simulink model "different_inverter_controls_BPS"  (R2024b)
settings: Solver=ode4  StartTime=0.0  StopTime=5  FixedStep=Ts  RelTol=1e-3
InitFcn:
  | %mode_of_operation=1;
  | %BESS_control_mode=1;
  | %Gen_Q_Control =1;
  | 
  | %Exciter_init;
  | 
  | %Exciter_init
  | Xq=0.474;
  | %%====================================================
  | % ST6C Exciter Parameters
  | 
  | KPA=30;
  | KIA=59.91;
  | KFF=1;
  | KM=1;
  | KLR=22.47;
  | KCL=1.04;
  | VAMAX=7.05;
  | VAMIN=-6.11;
  | VRMAX=7.05;
  | VRMIN=-6.11;
  | ILR=5.02;
  | KG=1;
  | TG=0.024;
  | TA=0.01;
  | VBMAX=999;
  | VMMAX=7.05;
  | VMMIN=-6.11;
  | KI=0;
  | Kp=1;
  | Kc=0;
  | Vt0=0;
  | VAAMAX=VAMAX;
  | %%========================================================
  | % UEL2C parameters
  | 
  | TUQ=.005;
  | TUP=0.050;
  | TUV=0.2;
  | TQREF=0;
  | Tadj=0;
  | K1=0;
  | K2=2;
  | VBIAS=1;
  | KFB=0;
  | TUL=0;
  | VUImax=1;
  | VUImin=-1;
  | VUELmax1=1;
  | VUELmax2=1;
  | VUELmin1=-1;
  | VUELmin2=-1;
  | KUF=0;
  | KUL=0.24;
  | KUI=0.001;
  | TU1=0;TU2=0;TU3=0;TU4=0;
  | KFIX=1;
  | VF=0;
  | VFB=0;
  | %%===========================================================
  | ... (+60 lines)
values from neighbouring files (symbols this model uses):
  inv1 = struct    [multiInverterParams.m]
  kp_sync = KQ_p/10    (= 0.04)    [multiInverterParams.m]
  Vdc = 1000    [multiInverterParams.m]
  Vpp = 480    [multiInverterParams.m]
undefined symbols (not defined in the file or in its folder): D1, Delta, DiscIntNeverNeededParam, Ion, Lithium, sigbuilder_block, sps
libraries: slpidlib x34, spsThreePhaseVIMeasurementLib x31, spsThreePhaseSeriesRLCBranchLib x23, spsabctodq0Lib x22, spsPower3phInstantaneousLib x22, spsThreePhaseTransformerTwoWindingsLib x16, spsSeriesRLCBranchLib x16, spsThreePhaseSeriesRLCLoadLib x14, simulink x12, spsPLL3phLib x11, spsGroundLib x9, powerlib_extras x8
(part 9 of 9)

== system different_inverter_controls_BPS/IBR-GFM Power Synchronization/Inverter/Power Controller/P,Q Control /Integrator1 ==
  w : Inport
  Constant1 : Constant  Commented=on  Value=2*pi  SampleTime=Ts
  Constant2 : Constant  Value=2*pi  SampleTime=Ts_Control
  Constant3 : Constant  Commented=on  Value=2*pi  SampleTime=Ts
  Constant4 : Constant  Commented=on  Value=f  SampleTime=Ts_Control
  Constant5 : Constant  Commented=on  Value=0  SampleTime=Ts_Control
  Discrete-Time Integrator : DiscreteIntegrator  Commented=on  IntegratorMethod=Integration: Trapezoidal  SampleTime=Ts  ICPrevOutput=DiscIntNeverNeededParam  ICPrevScaledInput=DiscIntNeverNeededParam
  Discrete-Time Integrator1 : DiscreteIntegrator  ExternalReset=rising  InitialConditionSource=external  SampleTime=Ts_Control  ShowStatePort=on  ICPrevOutput=DiscIntNeverNeededParam  ICPrevScaledInput=DiscIntNeverNeededParam
  Divide : Product  Commented=on  Inputs=*/
  From : From  Commented=on  GotoTag=fsys
  Gain : Gain  Commented=on  Gain=2*pi*f
  Gain1 : Gain  Commented=on  Gain=2*pi*f  SaturateOnIntegerOverflow=on  OutDataTypeStr=Inherit: Same as input  ParamDataTypeStr=Inherit: Same as input
  Gain3 : Gain  Gain=2*pi*f
  Hit Crossing : HitCross  Commented=on  HitCrossingOffset=pi  HitCrossingDirection=falling  ShowOutputPort=off
  Initial : InitialCondition  Value=0
  Initial1 : InitialCondition  Commented=on  Value=0
  Integrator : Integrator  Commented=on  ExternalReset=rising  InitialConditionSource=external  InitialCondition=sps.Phase_Init*pi/180  LimitOutput=on  ShowStatePort=on
  Integrator2 : Integrator  Commented=on  ExternalReset=rising  InitialConditionSource=external  InitialCondition=sps.Phase_Init*pi/180  ShowStatePort=on
  Math Function : Math  Commented=on  Operator=mod  SignedPower=on
  Relational Operator : RelationalOperator  Operator=>  OutDataTypeStr=boolean  InputSameDT=off
  Relational Operator1 : RelationalOperator  Commented=on  Operator=>  OutDataTypeStr=boolean  InputSameDT=off
  Scope : Scope
  Scope1 : Scope  Commented=on
  Scope2 : Scope  Commented=on
  Scope3 : Scope  Commented=on
  Subtract : Sum  Inputs=+-
  Subtract1 : Sum  Commented=on  Inputs=+-
  Sum1 : Sum  Commented=on  Inputs=|++
  Sum2 : Sum  Commented=on  Inputs=|+-
  Theta : Outport
  wires:
  Divide/1 -> Sum1/2
  Constant4/1 -> Divide/2
  From/1 -> Divide/1
  Sum2/1 -> Sum1/1, Scope2/1  "W"
  Constant5/1 -> Sum2/2
  Sum1/1 -> Gain/1  "W"
  Math Function/1 -> Scope1/1
  Constant3/1 -> Math Function/2
  Discrete-Time Integrator/1 -> Math Function/1
  Gain/1 -> Discrete-Time Integrator/1
  Discrete-Time Integrator1/1 -> Theta/1, Scope/1
  Subtract/1 -> Initial/1
  Constant2/1 -> Relational Operator/2, Subtract/2
  Discrete-Time Integrator1/State -> Relational Operator/1, Subtract/1
  Initial/1 -> Discrete-Time Integrator1/3
  Relational Operator/1 -> Discrete-Time Integrator1/2
  Subtract1/1 -> Initial1/1
  Integrator/1 -> Hit Crossing/1, Scope3/1
  Constant1/1 -> Relational Operator1/2, Subtract1/2
  Integrator/State -> Relational Operator1/1, Subtract1/1
  Relational Operator1/1 -> Integrator/2
  Initial1/1 -> Integrator/3
  Gain1/1 -> Integrator/1
  w/1 -> Gain3/1, Sum2/1
  Gain3/1 -> Discrete-Time Integrator1/1

== system different_inverter_controls_BPS/IBR-GFM Power Synchronization/Inverter/Power Controller/P,Q Control /Integrator2 ==
  w : Inport
  Constant1 : Constant  Commented=on  Value=2*pi  SampleTime=Ts
  Constant2 : Constant  Value=2*pi  SampleTime=Ts_Control
  Constant3 : Constant  Commented=on  Value=2*pi  SampleTime=Ts
  Constant4 : Constant  Commented=on  Value=f  SampleTime=Ts_Control
  Constant5 : Constant  Commented=on  Value=0  SampleTime=Ts_Control
  Discrete-Time Integrator : DiscreteIntegrator  Commented=on  IntegratorMethod=Integration: Trapezoidal  SampleTime=Ts  ICPrevOutput=DiscIntNeverNeededParam  ICPrevScaledInput=DiscIntNeverNeededParam
  Discrete-Time Integrator1 : DiscreteIntegrator  ExternalReset=rising  InitialConditionSource=external  SampleTime=Ts_Control  ShowStatePort=on  ICPrevOutput=DiscIntNeverNeededParam  ICPrevScaledInput=DiscIntNeverNeededParam
  Divide : Product  Commented=on  Inputs=*/
  From : From  Commented=on  GotoTag=fsys
  Gain : Gain  Commented=on  Gain=2*pi*f
  Gain1 : Gain  Commented=on  Gain=2*pi*f  SaturateOnIntegerOverflow=on  OutDataTypeStr=Inherit: Same as input  ParamDataTypeStr=Inherit: Same as input
  Gain3 : Gain  Gain=2*pi*f
  Hit Crossing : HitCross  Commented=on  HitCrossingOffset=pi  HitCrossingDirection=falling  ShowOutputPort=off
  Initial : InitialCondition  Value=0
  Initial1 : InitialCondition  Commented=on  Value=0
  Integrator : Integrator  Commented=on  ExternalReset=rising  InitialConditionSource=external  InitialCondition=sps.Phase_Init*pi/180  LimitOutput=on  ShowStatePort=on
  Integrator2 : Integrator  Commented=on  ExternalReset=rising  InitialConditionSource=external  InitialCondition=sps.Phase_Init*pi/180  ShowStatePort=on
  Math Function : Math  Commented=on  Operator=mod  SignedPower=on
  Relational Operator : RelationalOperator  Operator=>  OutDataTypeStr=boolean  InputSameDT=off
  Relational Operator1 : RelationalOperator  Commented=on  Operator=>  OutDataTypeStr=boolean  InputSameDT=off
  Scope : Scope
  Scope1 : Scope  Commented=on
  Scope2 : Scope  Commented=on
  Scope3 : Scope  Commented=on
  Subtract : Sum  Inputs=+-
  Subtract1 : Sum  Commented=on  Inputs=+-
  Sum1 : Sum  Commented=on  Inputs=|++
  Sum2 : Sum  Commented=on  Inputs=|+-
  Theta : Outport
  wires:
  Gain3/1 -> Discrete-Time Integrator1/1
  w/1 -> Sum2/1, Gain3/1
  Gain1/1 -> Integrator/1
  Initial1/1 -> Integrator/3
  Relational Operator1/1 -> Integrator/2
  Integrator/State -> Subtract1/1, Relational Operator1/1
  Constant1/1 -> Subtract1/2, Relational Operator1/2
  Integrator/1 -> Scope3/1, Hit Crossing/1
  Subtract1/1 -> Initial1/1
  Relational Operator/1 -> Discrete-Time Integrator1/2
  Initial/1 -> Discrete-Time Integrator1/3
  Discrete-Time Integrator1/State -> Subtract/1, Relational Operator/1
  Constant2/1 -> Subtract/2, Relational Operator/2
  Subtract/1 -> Initial/1
  Discrete-Time Integrator1/1 -> Scope/1, Theta/1
  Gain/1 -> Discrete-Time Integrator/1
  Discrete-Time Integrator/1 -> Math Function/1
  Constant3/1 -> Math Function/2
  Math Function/1 -> Scope1/1
  Sum1/1 -> Gain/1  "W"
  Constant5/1 -> Sum2/2
  Sum2/1 -> Scope2/1, Sum1/1  "W"
  From/1 -> Divide/1
  Constant4/1 -> Divide/2
  Divide/1 -> Sum1/2

== system different_inverter_controls_BPS/GFM-VSG-100MW/IBR-GFM VSG/Inverter/Inverter Control/Current Control/Current Regulator ==
  note: Current Regulator
      | ================
  note: Sign Convention: Current going out of the converter = positive current
  note: Iq positive --> The converter absorbs reactive power ("Inductive mode") = Reactive Power Q negative
  note: Id positive --> The converter generates active power ("Inverter mode") = Active Power P positive
  VdVq_meas : Inport  PortDimensions=2
  IdIq_meas : Inport  Port=2  PortDimensions=2
  IdIq_ref : Inport  Port=3  PortDimensions=2
  Add1 : Sum  Inputs=++-
  Add2 : Sum
  Add3 : Sum  Inputs=+++
  Demux : Demux  Outputs=2
  Demux1 : Demux  Outputs=2
  Lff : Gain  Gain=inv1.Lpu  SaturateOnIntegerOverflow=on  OutDataTypeStr=Inherit: Same as input  ParamDataTypeStr=Inherit: Same as input
  "Lff  " : Gain  Gain=inv1.Lpu  SaturateOnIntegerOverflow=on  OutDataTypeStr=Inherit: Same as input  ParamDataTypeStr=Inherit: Same as input
  Lff  1 : Gain  Commented=on  Gain=Ltot_pu  SaturateOnIntegerOverflow=on  OutDataTypeStr=Inherit: Same as input  ParamDataTypeStr=Inherit: Same as input
  Mux : Mux  Inputs=2
  PI : slpidlib/PID Controller  Controller=PI  Form=Parallel  TimeDomain=Discrete-time  UseExternalTs=off  SampleTime=Ts_Control  IntegratorMethod=Forward Euler  FilterMethod=Forward Euler  ControllerParametersSource=internal  P=Kp_Ireg/10  I=Ki_Ireg  UseKiTs=off  D=0  UseExternalDerivativeSource=off  N=100  UseFilter=on  TunerSelectOption=Transfer Function Based (PID Tuner App)  InitialConditionSource=internal  InitialConditionForIntegrator=0  InitialConditionForFilter=0  DifferentiatorICPrevScaledInput=0  ExternalReset=none  TrackingMode=off  Kt=1  LimitOutput=on  SatLimitsSource=internal  UpperSaturationLimit=1.5  LowerSaturationLimit=-1.5  LinearizeAsGain=off  AntiWindupMode=back-calculation  Kb=1  LimitIntegrator=off  UpperIntegratorSaturationLimit=inf  LowerIntegratorSaturationLimit=-inf  POutMin=[]  POutMax=[]  IOutMin=[]  IOutMax=[]  DOutMin=[]  DOutMax=[]  NOutMin=[]  NOutMax=[]  SumOutMin=[]  SumOutMax=[]  SaturationOutMin=[]  SaturationOutMax=[]  PParamMin=[]  PParamMax=[]  IParamMin=[]  IParamMax=[]  DParamMin=[]  DParamMax=[]  NParamMin=[]  NParamMax=[]  KbParamMin=[]  KbParamMax=[]  KtParamMin=[]  KtParamMax=[]  KbOutMin=[]  KbOutMax=[]  KtOutMin=[]  KtOutMax=[]  IntegratorOutMin=[]  IntegratorOutMax=[]  FilterOutMin=[]  FilterOutMax=[]  SumI1OutMin=[]  SumI1OutMax=[]  SumI2OutMin=[]  SumI2OutMax=[]  SumI3OutMin=[]  SumI3OutMax=[]  SumI4OutMin=[]  SumI4OutMax=[]  SumDOutMin=[]  SumDOutMax=[]  DifferentiatorOutMin=[]  DifferentiatorOutMax=[]  FilterDiffOutCoefMin=[]  FilterDiffOutCoefMax=[]  ReciprocalOutMin=[]  ReciprocalOutMax=[]  SumDenOutMin=[]  SumDenOutMax=[]  SumNumOutMin=[]  SumNumOutMax=[]  DivideOutMin=[]  DivideOutMax=[]  UdiffTsProdOutMin=[]  UdiffTsProdOutMax=[]  NTsProdOutMin=[]  NTsProdOutMax=[]  UintegralTsProdOutMin=[]  UintegralTsProdOutMax=[]  UngainTsProdOutMin=[]  UngainTsProdOutMax=[]  ClampingZeroOutDataTypeStr=Inherit: Inherit via back propagation  ClampingZeroOutMin=[]  ClampingZeroOutMax=[]  FilterDenConstantOutDataTypeStr=Inherit: Inherit via back propagation  FilterDenConstantOutMin=[]  FilterDenConstantOutMax=[]  PCopyOutDataTypeStr=Inherit: Inherit via back propagation  PCopyOutMin=[]  PCopyOutMax=[]  NCopyOutDataTypeStr=Inherit: Inherit via back propagation  NCopyOutMin=[]  NCopyOutMax=[]  IntegratorContinuousStateAttributes=''  IntegratorStateMustResolveToSignalObject=off  IntegratorRTWStateStorageClass=Auto  FilterContinuousStateAttributes=''  FilterStateMustResolveToSignalObject=off  FilterRTWStateStorageClass=Auto  ParallelPVariant=InternalParameters  IdealPVariant=Disabled  IVariant=InternalParameters  DVariant=Disabled  IntegratorVariant=Discrete  SatVariant=Enabled  AWVariant=BackCalculation  PCopyVariant=Disabled  TRVariant=Disabled  FdbkBlocksVariant=Forward  IdealPFdbkVariant=Disabled  SatFdbkVariant=Disabled  DerivativeFilterVariant=Disabled  NVariant=Disabled  NCopyVariant=Disabled_SignalSpec  FilterICVariant=Disabled  IntegratorICVariant=InternalICs  ExternalResetVariant=Disabled  TRSumVariant=Passthrough  SumFdbkVariant=Disabled  SumVariant=Sum_PI  TsampFilterVariant=InternalTs  TsampNgainVariant=Passthrough  TsampIntegralVariant=Disabled_SignalSpec  ExternalSaturationOutDataTypeStr=Inherit: Same as second input  DerivativeSourceVariant=Disabled  PreIntVariant=InternalPreInt
  PI1 : slpidlib/PID Controller  Commented=on  Controller=PI  Form=Parallel  TimeDomain=Discrete-time  UseExternalTs=off  SampleTime=Ts_Control  IntegratorMethod=Forward Euler  FilterMethod=Forward Euler  ControllerParametersSource=internal  P=Kp_Ireg  I=Ki_Ireg  UseKiTs=off  D=0  UseExternalDerivativeSource=off  N=100  UseFilter=on  TunerSelectOption=Transfer Function Based (PID Tuner App)  InitialConditionSource=internal  InitialConditionForIntegrator=0  InitialConditionForFilter=0  DifferentiatorICPrevScaledInput=0  ExternalReset=none  TrackingMode=off  Kt=1  LimitOutput=on  SatLimitsSource=internal  UpperSaturationLimit=1.5  LowerSaturationLimit=-1.5  LinearizeAsGain=off  AntiWindupMode=clamping  Kb=1  LimitIntegrator=off  UpperIntegratorSaturationLimit=inf  LowerIntegratorSaturationLimit=-inf  POutMin=[]  POutMax=[]  IOutMin=[]  IOutMax=[]  DOutMin=[]  DOutMax=[]  NOutMin=[]  NOutMax=[]  SumOutMin=[]  SumOutMax=[]  SaturationOutMin=[]  SaturationOutMax=[]  PParamMin=[]  PParamMax=[]  IParamMin=[]  IParamMax=[]  DParamMin=[]  DParamMax=[]  NParamMin=[]  NParamMax=[]  KbParamMin=[]  KbParamMax=[]  KtParamMin=[]  KtParamMax=[]  KbOutMin=[]  KbOutMax=[]  KtOutMin=[]  KtOutMax=[]  IntegratorOutMin=[]  IntegratorOutMax=[]  FilterOutMin=[]  FilterOutMax=[]  SumI1OutMin=[]  SumI1OutMax=[]  SumI2OutMin=[]  SumI2OutMax=[]  SumI3OutMin=[]  SumI3OutMax=[]  SumI4OutMin=[]  SumI4OutMax=[]  SumDOutMin=[]  SumDOutMax=[]  DifferentiatorOutMin=[]  DifferentiatorOutMax=[]  FilterDiffOutCoefMin=[]  FilterDiffOutCoefMax=[]  ReciprocalOutMin=[]  ReciprocalOutMax=[]  SumDenOutMin=[]  SumDenOutMax=[]  SumNumOutMin=[]  SumNumOutMax=[]  DivideOutMin=[]  DivideOutMax=[]  UdiffTsProdOutMin=[]  UdiffTsProdOutMax=[]  NTsProdOutMin=[]  NTsProdOutMax=[]  UintegralTsProdOutMin=[]  UintegralTsProdOutMax=[]  UngainTsProdOutMin=[]  UngainTsProdOutMax=[]  ClampingZeroOutDataTypeStr=Inherit: Inherit via back propagation  ClampingZeroOutMin=[]  ClampingZeroOutMax=[]  FilterDenConstantOutDataTypeStr=Inherit: Inherit via back propagation  FilterDenConstantOutMin=[]  FilterDenConstantOutMax=[]  PCopyOutDataTypeStr=Inherit: Inherit via back propagation  PCopyOutMin=[]  PCopyOutMax=[]  NCopyOutDataTypeStr=Inherit: Inherit via back propagation  NCopyOutMin=[]  NCopyOutMax=[]  IntegratorContinuousStateAttributes=''  IntegratorStateMustResolveToSignalObject=off  IntegratorRTWStateStorageClass=Auto  FilterContinuousStateAttributes=''  FilterStateMustResolveToSignalObject=off  FilterRTWStateStorageClass=Auto  ParallelPVariant=InternalParameters  IdealPVariant=Disabled  IVariant=InternalParameters  DVariant=Disabled  IntegratorVariant=Discrete  SatVariant=Enabled  AWVariant=DiscClampingParallel  PCopyVariant=Disabled  TRVariant=Disabled  FdbkBlocksVariant=Forward  IdealPFdbkVariant=Disabled  SatFdbkVariant=Disabled  DerivativeFilterVariant=Disabled  NVariant=Disabled  NCopyVariant=Disabled_SignalSpec  FilterICVariant=Disabled  IntegratorICVariant=InternalICs  ExternalResetVariant=Disabled  TRSumVariant=Passthrough  SumFdbkVariant=Disabled  SumVariant=Sum_PI  TsampFilterVariant=InternalTs  TsampNgainVariant=Passthrough  TsampIntegralVariant=Disabled_SignalSpec  ExternalSaturationOutDataTypeStr=Inherit: Same as second input  DerivativeSourceVariant=Disabled  PreIntVariant=InternalPreInt
  PI2 : slpidlib/PID Controller  Commented=on  Controller=PI  Form=Parallel  TimeDomain=Discrete-time  UseExternalTs=off  SampleTime=Ts_Control  IntegratorMethod=Forward Euler  FilterMethod=Forward Euler  ControllerParametersSource=internal  P=Kp_Ireg  I=Ki_Ireg  UseKiTs=off  D=0  UseExternalDerivativeSource=off  N=100  UseFilter=on  TunerSelectOption=Transfer Function Based (PID Tuner App)  InitialConditionSource=internal  InitialConditionForIntegrator=0  InitialConditionForFilter=0  DifferentiatorICPrevScaledInput=0  ExternalReset=none  TrackingMode=off  Kt=1  LimitOutput=on  SatLimitsSource=internal  UpperSaturationLimit=1.5  LowerSaturationLimit=-1.5  LinearizeAsGain=off  AntiWindupMode=back-calculation  Kb=1  LimitIntegrator=off  UpperIntegratorSaturationLimit=inf  LowerIntegratorSaturationLimit=-inf  POutMin=[]  POutMax=[]  IOutMin=[]  IOutMax=[]  DOutMin=[]  DOutMax=[]  NOutMin=[]  NOutMax=[]  SumOutMin=[]  SumOutMax=[]  SaturationOutMin=[]  SaturationOutMax=[]  PParamMin=[]  PParamMax=[]  IParamMin=[]  IParamMax=[]  DParamMin=[]  DParamMax=[]  NParamMin=[]  NParamMax=[]  KbParamMin=[]  KbParamMax=[]  KtParamMin=[]  KtParamMax=[]  KbOutMin=[]  KbOutMax=[]  KtOutMin=[]  KtOutMax=[]  IntegratorOutMin=[]  IntegratorOutMax=[]  FilterOutMin=[]  FilterOutMax=[]  SumI1OutMin=[]  SumI1OutMax=[]  SumI2OutMin=[]  SumI2OutMax=[]  SumI3OutMin=[]  SumI3OutMax=[]  SumI4OutMin=[]  SumI4OutMax=[]  SumDOutMin=[]  SumDOutMax=[]  DifferentiatorOutMin=[]  DifferentiatorOutMax=[]  FilterDiffOutCoefMin=[]  FilterDiffOutCoefMax=[]  ReciprocalOutMin=[]  ReciprocalOutMax=[]  SumDenOutMin=[]  SumDenOutMax=[]  SumNumOutMin=[]  SumNumOutMax=[]  DivideOutMin=[]  DivideOutMax=[]  UdiffTsProdOutMin=[]  UdiffTsProdOutMax=[]  NTsProdOutMin=[]  NTsProdOutMax=[]  UintegralTsProdOutMin=[]  UintegralTsProdOutMax=[]  UngainTsProdOutMin=[]  UngainTsProdOutMax=[]  ClampingZeroOutDataTypeStr=Inherit: Inherit via back propagation  ClampingZeroOutMin=[]  ClampingZeroOutMax=[]  FilterDenConstantOutDataTypeStr=Inherit: Inherit via back propagation  FilterDenConstantOutMin=[]  FilterDenConstantOutMax=[]  PCopyOutDataTypeStr=Inherit: Inherit via back propagation  PCopyOutMin=[]  PCopyOutMax=[]  NCopyOutDataTypeStr=Inherit: Inherit via back propagation  NCopyOutMin=[]  NCopyOutMax=[]  IntegratorContinuousStateAttributes=''  IntegratorStateMustResolveToSignalObject=off  IntegratorRTWStateStorageClass=Auto  FilterContinuousStateAttributes=''  FilterStateMustResolveToSignalObject=off  FilterRTWStateStorageClass=Auto  ParallelPVariant=InternalParameters  IdealPVariant=Disabled  IVariant=InternalParameters  DVariant=Disabled  IntegratorVariant=Discrete  SatVariant=Enabled  AWVariant=BackCalculation  PCopyVariant=Disabled  TRVariant=Disabled  FdbkBlocksVariant=Forward  IdealPFdbkVariant=Disabled  SatFdbkVariant=Disabled  DerivativeFilterVariant=Disabled  NVariant=Disabled  NCopyVariant=Disabled_SignalSpec  FilterICVariant=Disabled  IntegratorICVariant=InternalICs  ExternalResetVariant=Disabled  TRSumVariant=Passthrough  SumFdbkVariant=Disabled  SumVariant=Sum_PI  TsampFilterVariant=InternalTs  TsampNgainVariant=Passthrough  TsampIntegralVariant=Disabled_SignalSpec  ExternalSaturationOutDataTypeStr=Inherit: Same as second input  DerivativeSourceVariant=Disabled  PreIntVariant=InternalPreInt
  Rff : Gain  Commented=on  Gain=inv1.R/inv1.Zb  SaturateOnIntegerOverflow=on  OutDataTypeStr=Inherit: Same as input  ParamDataTypeStr=Inherit: Same as input
  "Rff " : Gain  Commented=on  Gain=inv1.R/inv1.Zb  SaturateOnIntegerOverflow=on  OutDataTypeStr=Inherit: Same as input  ParamDataTypeStr=Inherit: Same as input
  Rff 1 : Gain  Commented=on  Gain=Rtot_pu  SaturateOnIntegerOverflow=on  OutDataTypeStr=Inherit: Same as input  ParamDataTypeStr=Inherit: Same as input
  Saturation : Saturate  UpperLimit=1.5  LowerLimit=-1.5
  Scope : Scope  NumInputPorts=2
  Scope1 : Scope
  Sum : Sum  Inputs=|-+
  VdVq_conv : Outport  VectorParamsAs1DForOutWhenUnconnected=off
  wires:
  Mux/1 -> Add2/2
  PI/1 -> Scope/2, Add2/1  "PI"
  Sum/1 -> Scope/1, PI/1
  IdIq_ref/1 -> Sum/2
  IdIq_meas/1 -> Demux1/1, Sum/1
  Add2/1 -> Saturation/1
  Saturation/1 -> Scope1/1, VdVq_conv/1
  VdVq_meas/1 -> Demux/1
  Demux/1 -> Add1/1
  "Rff "/1 -> Add1/2
  Demux1/1 -> "Rff "/1, Lff/1
  "Lff  "/1 -> Add1/3
  Demux1/2 -> "Lff  "/1, Rff/1
  Rff/1 -> Add3/2
  Lff/1 -> Add3/3
  Add1/1 -> Mux/1  "Feedforward"
  Demux/2 -> Add3/1
  Add3/1 -> Mux/2

== system different_inverter_controls_BPS/GFM-VSG-100MW/IBR-GFM VSG/Inverter/Inverter Control/Current Control/Uabc_ref Generation max (m) = 1 ==
  note: (Correction for transformer
      |  D1 connection)
  note: (Correction for delay of Ts_Control)
  note: Uref Generation
      | ==============
  wt : Inport
  VdVq_conv : Inport  Port=2
  Add1 : Sum  Inputs=++++
  Add2 : Sum
  Complex to Magnitude-Angle : ComplexToMagnitudeAngle
  Constant : Constant  Commented=on  Value=-pi/6
  Constant1 : Constant  Commented=on  Value=Vnom_dc
  Constant2 : Constant  Value="[ 0  -2*pi/3  2*pi/3  ]"
  Constant3 : Constant  Commented=on  Value=Vnom_sec*sqrt(2)/sqrt(3)
  Constant4 : Constant  Value=Ts_Control*Fnom*(2*pi)
  Constant5 : Constant  Value=Vdc
  Constant6 : Constant  Value=Vpp*sqrt(2)/sqrt(3)
  Demux1 : Demux  Outputs=2
  Gain1 : Gain  Gain=1/2
  Product : Product  Inputs=*/  RndMeth=Zero
  Product1 : Product  Inputs=*/  RndMeth=Zero
  Product2 : Product  Inputs=**  RndMeth=Zero
  Real-Imag to Complex : RealImagToComplex
  Trigonometric Function : Trigonometry
  Uabc_ref : Outport  VectorParamsAs1DForOutWhenUnconnected=off
  wires:
  Constant5/1 -> Gain1/1
  VdVq_conv/1 -> Product1/1
  Product1/1 -> Demux1/1
  Gain1/1 -> Product/1
  Real-Imag to Complex/1 -> Complex to Magnitude-Angle/1
  Demux1/1 -> Real-Imag to Complex/1
  Demux1/2 -> Real-Imag to Complex/2
  Constant2/1 -> Add1/2
  Constant/1 -> Add1/3
  Constant6/1 -> Product/2
  Complex to Magnitude-Angle/2 -> Add2/1
  Add1/1 -> Add2/2
  Add2/1 -> Trigonometric Function/1
  Complex to Magnitude-Angle/1 -> Product2/1
  Trigonometric Function/1 -> Product2/2
  Product2/1 -> Uabc_ref/1
  wt/1 -> Add1/1
  Constant4/1 -> Add1/4
  Product/1 -> Product1/2

== system different_inverter_controls_BPS/GFM-VSG-100MW/IBR-GFM VSG/Inverter/Inverter Control/current limiter/P priority limit ==
  idiqP : Inport
  Demux4 : Demux  Outputs=2
  IqLimit : Subsystem
  Mux4 : Mux  Inputs=2
  Rtot_pu1 : Gain  Gain=-1  SaturateOnIntegerOverflow=on  OutDataTypeStr=Inherit: Same as input  ParamDataTypeStr=Inherit: Same as input
  Saturation : Saturate  UpperLimit=limMax  LowerLimit=0
  Saturation Dynamic : simulink/Discontinuities/Saturation Dynamic  OutMin=[]  OutMax=[limMax]  OutDataTypeStr=Inherit: Same as second input  OutDataType=fixdt(1, 16)  OutScaling=2^-10  DoSatur=off
  idiqPRefL : Outport
  wires:
  IqLimit/1(Out2) -> Saturation Dynamic/1, Rtot_pu1/1
  Rtot_pu1/1 -> Saturation Dynamic/3
  Saturation/1 -> Mux4/1, IqLimit/1(In1)
  Demux4/1 -> Saturation/1
  Mux4/1 -> idiqPRefL/1
  Demux4/2 -> Saturation Dynamic/2
  idiqP/1 -> Demux4/1
  Saturation Dynamic/1 -> Mux4/2

== system different_inverter_controls_BPS/GFM-VSG-100MW/IBR-GFM VSG/Inverter/Inverter Control/current limiter/Q priority limit ==
  idiqP : Inport
  V_inv_mag : Inport  Port=2
  Demux4 : Demux  Outputs=2
  Iq condition : Switch  Threshold=0.9  SaturateOnIntegerOverflow=off  InputSameDT=off
  IqLimit : Subsystem
  Mux4 : Mux  Inputs=2
  Rtot_pu1 : Gain  Gain=-1  SaturateOnIntegerOverflow=on  OutDataTypeStr=Inherit: Same as input  ParamDataTypeStr=Inherit: Same as input
  Saturation : Saturate  UpperLimit=limMax  LowerLimit=limMin
  Saturation Dynamic : simulink/Discontinuities/Saturation Dynamic  OutMin=[]  OutMax=[]  OutDataTypeStr=Inherit: Same as second input  OutDataType=fixdt(1, 16)  OutScaling=2^-10  DoSatur=off
  Saturation1 : Saturate  UpperLimit=0  LowerLimit=limMin
  Scope : Scope
  idiqPRefL : Outport
  wires:
  Demux4/2 -> Saturation1/1, Saturation/1
  Saturation1/1 -> Iq condition/3
  IqLimit/1(Out2) -> Saturation Dynamic/1, Rtot_pu1/1
  Demux4/1 -> Saturation Dynamic/2
  Saturation Dynamic/1 -> Mux4/1
  Rtot_pu1/1 -> Saturation Dynamic/3
  Mux4/1 -> idiqPRefL/1
  idiqP/1 -> Demux4/1
  Saturation/1 -> Iq condition/1
  V_inv_mag/1 -> Iq condition/2
  Iq condition/1 -> IqLimit/1(In1), Mux4/2

== system different_inverter_controls_BPS/GFM-VSG-100MW/IBR-GFM VSG/Inverter/Inverter Control/current limiter/Subsystem3 ==
  In1 : Inport
  Demux2 : Demux  Outputs=2
  Math Function : Math  Operator=square  SignedPower=on
  Saturation : Saturate  UpperLimit=limMax  LowerLimit=limMin
  Scope : Scope  NumInputPorts=2
  Sqrt1 : Sqrt
  Subtract : Sum
  Out1 : Outport
  Out2 : Outport  Port=2
  wires:
  Saturation/1 -> Out1/1
  Sqrt1/1 -> Out2/1, Scope/1, Saturation/1
  Subtract/1 -> Sqrt1/1  "Ipos2"
  In1/1 -> Math Function/1, Scope/2
  Math Function/1 -> Demux2/1
  Demux2/1 -> Subtract/1
  Demux2/2 -> Subtract/2

== system different_inverter_controls_BPS/GFM-VSG-100MW/IBR-GFM VSG/Inverter/Inverter Control/current limiter/Subsystem4 ==
  In1 : Inport
  In2 : Inport  Port=2
  Demux4 : Demux  Outputs=2
  Mux4 : Mux  Inputs=2
  Switch1 : Switch  Threshold=limMax  SaturateOnIntegerOverflow=off  InputSameDT=off
  Unit Delay2 : UnitDelay  InitialCondition=1  SampleTime=Ts_Control  HasFrameUpgradeWarning=on
  dummy limit : Saturate  UpperLimit=limMax  LowerLimit=limMin
  Out1 : Outport
  wires:
  dummy limit/1 -> Mux4/2
  Demux4/2 -> dummy limit/1
  In2/1 -> Demux4/1, Switch1/3
  In1/1 -> Switch1/2
  Unit Delay2/1 -> Switch1/1
  Switch1/1 -> Unit Delay2/1, Mux4/1, Out1/1

== system different_inverter_controls_BPS/GFM-VSG-100MW/IBR-GFM VSG/Inverter/Inverter Control/current limiter/Subsystem9 ==
  In1 : Inport
  In2 : Inport  Port=2
  Divide : Product  Inputs=*/
  Gain1 : Gain  Gain=limMax
  Saturation : Saturate  UpperLimit=limMax  LowerLimit=limMin
  Switch1 : Switch  Threshold=limMax  SaturateOnIntegerOverflow=off  InputSameDT=off
  idiqPRefL : Outport
  wires:
  Saturation/1 -> idiqPRefL/1
  Switch1/1 -> Saturation/1
  Gain1/1 -> Switch1/1
  Divide/1 -> Gain1/1
  In2/1 -> Switch1/3, Divide/1
  In1/1 -> Switch1/2, Divide/2

== system different_inverter_controls_BPS/GFM-VSG-100MW/IBR-GFM VSG/Inverter/Power Controller/P,Q Control /Integrator ==
  w : Inport
  Constant2 : Constant  Value=2*pi  SampleTime=Ts_Control
  Discrete-Time Integrator1 : DiscreteIntegrator  ExternalReset=rising  InitialConditionSource=external  SampleTime=Ts_Control  ShowStatePort=on  ICPrevOutput=DiscIntNeverNeededParam  ICPrevScaledInput=DiscIntNeverNeededParam
  Gain3 : Gain  Gain=2*pi*f
  Initial : InitialCondition  Value=0
  Relational Operator : RelationalOperator  Operator=>  OutDataTypeStr=boolean  InputSameDT=off
  Scope : Scope
  Subtract : Sum  Inputs=+-
  Theta : Outport
  wires:
  Discrete-Time Integrator1/1 -> Theta/1, Scope/1
  Subtract/1 -> Initial/1
  Constant2/1 -> Relational Operator/2, Subtract/2
  Discrete-Time Integrator1/State -> Relational Operator/1, Subtract/1
  Initial/1 -> Discrete-Time Integrator1/3
  Relational Operator/1 -> Discrete-Time Integrator1/2
  w/1 -> Gain3/1
  Gain3/1 -> Discrete-Time Integrator1/1

== system different_inverter_controls_BPS/IBR GFL-SH/BESS/Inverter Control/current limiter/P priority limit/IqLimit ==
  In1 : Inport
  Math Function : Math  Operator=square  SignedPower=on
  Math Function1 : Math  Operator=square  SignedPower=on
  Sqrt : Sqrt
  Subtract : Sum  Inputs=+-
  Vdc_ref1 : Constant  Value=limMax  SampleTime=Ts_Control
  Out2 : Outport
  wires:
  Math Function1/1 -> Subtract/2
  In1/1 -> Math Function1/1
  Vdc_ref1/1 -> Math Function/1
  Subtract/1 -> Sqrt/1
  Sqrt/1 -> Out2/1
  Math Function/1 -> Subtract/1

== system different_inverter_controls_BPS/IBR GFL-SH/BESS/Inverter Control/current limiter/Q priority limit/IqLimit ==
  In1 : Inport
  Math Function : Math  Operator=square  SignedPower=on
  Math Function1 : Math  Operator=square  SignedPower=on
  Sqrt : Sqrt
  Subtract : Sum  Inputs=+-
  Vdc_ref1 : Constant  Value=limMax  SampleTime=Ts_Control
  Out2 : Outport
  wires:
  Math Function1/1 -> Subtract/2
  In1/1 -> Math Function1/1
  Vdc_ref1/1 -> Math Function/1
  Subtract/1 -> Sqrt/1
  Sqrt/1 -> Out2/1
  Math Function/1 -> Subtract/1

== system different_inverter_controls_BPS/IBR GFL-SH/IBR/Inverter Control/current limiter/P priority limit/IqLimit ==
  In1 : Inport
  Math Function : Math  Operator=square  SignedPower=on
  Math Function1 : Math  Operator=square  SignedPower=on
  Sqrt : Sqrt
  Subtract : Sum  Inputs=+-
  Vdc_ref1 : Constant  Value=limMax  SampleTime=Ts_Control
  Out2 : Outport
  wires:
  Math Function1/1 -> Subtract/2
  In1/1 -> Math Function1/1
  Vdc_ref1/1 -> Math Function/1
  Subtract/1 -> Sqrt/1
  Sqrt/1 -> Out2/1
  Math Function/1 -> Subtract/1

== system different_inverter_controls_BPS/IBR GFL-SH/IBR/Inverter Control/current limiter/Q priority limit/IqLimit ==
  In1 : Inport
  Math Function : Math  Operator=square  SignedPower=on
  Math Function1 : Math  Operator=square  SignedPower=on
  Sqrt : Sqrt
  Subtract : Sum  Inputs=+-
  Vdc_ref1 : Constant  Value=limMax  SampleTime=Ts_Control
  Out2 : Outport
  wires:
  Math Function1/1 -> Subtract/2
  In1/1 -> Math Function1/1
  Vdc_ref1/1 -> Math Function/1
  Subtract/1 -> Sqrt/1
  Sqrt/1 -> Out2/1
  Math Function/1 -> Subtract/1

== system different_inverter_controls_BPS/IBR-GFM PV Droop/IBR/Inverter Control/current limiter/P priority limit/IqLimit ==
  In1 : Inport
  Math Function : Math  Operator=square  SignedPower=on
  Math Function1 : Math  Operator=square  SignedPower=on
  Sqrt : Sqrt
  Subtract : Sum  Inputs=+-
  Vdc_ref1 : Constant  Value=limMax  SampleTime=Ts_Control
  Out2 : Outport
  wires:
  Math Function1/1 -> Subtract/2
  In1/1 -> Math Function1/1
  Vdc_ref1/1 -> Math Function/1
  Subtract/1 -> Sqrt/1
  Sqrt/1 -> Out2/1
  Math Function/1 -> Subtract/1

== system different_inverter_controls_BPS/IBR-GFM PV Droop/IBR/Inverter Control/current limiter/Q priority limit/IqLimit ==
  In1 : Inport
  Math Function : Math  Operator=square  SignedPower=on
  Math Function1 : Math  Operator=square  SignedPower=on
  Sqrt : Sqrt
  Subtract : Sum  Inputs=+-
  Vdc_ref1 : Constant  Value=limMax  SampleTime=Ts_Control
  Out2 : Outport
  wires:
  Math Function1/1 -> Subtract/2
  In1/1 -> Math Function1/1
  Vdc_ref1/1 -> Math Function/1
  Subtract/1 -> Sqrt/1
  Sqrt/1 -> Out2/1
  Math Function/1 -> Subtract/1

== system different_inverter_controls_BPS/IBR-GFM Synchro-inverter/Inverter/Inverter Control/current limiter/P priority limit/IqLimit ==
  In1 : Inport
  Math Function : Math  Operator=square  SignedPower=on
  Math Function1 : Math  Operator=square  SignedPower=on
  Sqrt : Sqrt
  Subtract : Sum  Inputs=+-
  Vdc_ref1 : Constant  Value=limMax  SampleTime=Ts_Control
  Out2 : Outport
  wires:
  Math Function/1 -> Subtract/1
  Sqrt/1 -> Out2/1
  Subtract/1 -> Sqrt/1
  Vdc_ref1/1 -> Math Function/1
  In1/1 -> Math Function1/1
  Math Function1/1 -> Subtract/2

== system different_inverter_controls_BPS/IBR-GFM Synchro-inverter/Inverter/Inverter Control/current limiter/Q priority limit/IqLimit ==
  In1 : Inport
  Math Function : Math  Operator=square  SignedPower=on
  Math Function1 : Math  Operator=square  SignedPower=on
  Sqrt : Sqrt
  Subtract : Sum  Inputs=+-
  Vdc_ref1 : Constant  Value=limMax  SampleTime=Ts_Control
  Out2 : Outport
  wires:
  Math Function/1 -> Subtract/1
  Sqrt/1 -> Out2/1
  Subtract/1 -> Sqrt/1
  Vdc_ref1/1 -> Math Function/1
  In1/1 -> Math Function1/1
  Math Function1/1 -> Subtract/2

== system different_inverter_controls_BPS/IBR-GFM Power Synchronization/Inverter/Inverter Control/current limiter/P priority limit/IqLimit ==
  In1 : Inport
  Math Function : Math  Operator=square  SignedPower=on
  Math Function1 : Math  Operator=square  SignedPower=on
  Sqrt : Sqrt
  Subtract : Sum  Inputs=+-
  Vdc_ref1 : Constant  Value=limMax  SampleTime=Ts_Control
  Out2 : Outport
  wires:
  Math Function/1 -> Subtract/1
  Sqrt/1 -> Out2/1
  Subtract/1 -> Sqrt/1
  Vdc_ref1/1 -> Math Function/1
  In1/1 -> Math Function1/1
  Math Function1/1 -> Subtract/2

== system different_inverter_controls_BPS/IBR-GFM Power Synchronization/Inverter/Inverter Control/current limiter/Q priority limit/IqLimit ==
  In1 : Inport
  Math Function : Math  Operator=square  SignedPower=on
  Math Function1 : Math  Operator=square  SignedPower=on
  Sqrt : Sqrt
  Subtract : Sum  Inputs=+-
  Vdc_ref1 : Constant  Value=limMax  SampleTime=Ts_Control
  Out2 : Outport
  wires:
  Math Function/1 -> Subtract/1
  Sqrt/1 -> Out2/1
  Subtract/1 -> Sqrt/1
  Vdc_ref1/1 -> Math Function/1
  In1/1 -> Math Function1/1
  Math Function1/1 -> Subtract/2

== system different_inverter_controls_BPS/GFM-VSG-100MW/IBR-GFM VSG/Inverter/Inverter Control/current limiter/P priority limit/IqLimit ==
  In1 : Inport
  Math Function : Math  Operator=square  SignedPower=on
  Math Function1 : Math  Operator=square  SignedPower=on
  Sqrt : Sqrt
  Subtract : Sum  Inputs=+-
  Vdc_ref1 : Constant  Value=limMax  SampleTime=Ts_Control
  Out2 : Outport
  wires:
  Math Function1/1 -> Subtract/2
  In1/1 -> Math Function1/1
  Vdc_ref1/1 -> Math Function/1
  Subtract/1 -> Sqrt/1
  Sqrt/1 -> Out2/1
  Math Function/1 -> Subtract/1

== system different_inverter_controls_BPS/GFM-VSG-100MW/IBR-GFM VSG/Inverter/Inverter Control/current limiter/Q priority limit/IqLimit ==
  In1 : Inport
  Math Function : Math  Operator=square  SignedPower=on
  Math Function1 : Math  Operator=square  SignedPower=on
  Sqrt : Sqrt
  Subtract : Sum  Inputs=+-
  Vdc_ref1 : Constant  Value=limMax  SampleTime=Ts_Control
  Out2 : Outport
  wires:
  Math Function1/1 -> Subtract/2
  In1/1 -> Math Function1/1
  Vdc_ref1/1 -> Math Function/1
  Subtract/1 -> Sqrt/1
  Sqrt/1 -> Out2/1
  Math Function/1 -> Subtract/1

== matlab function different_inverter_controls_BPS/GFM-VSG-100MW/FRT/In -RSY/dTheta calc ==
  data: in input; out output
function out  = fcn(in)
    persistent cnt inOld flag outOld
    if isempty(cnt)
        cnt = 1;
    end
    if isempty(inOld)
        inOld = 0;
    end 
    if isempty(flag)
        flag = 0;
    end
    if isempty(outOld)
        outOld = 0;
    end    
out = outOld;
temp = in - inOld; 

if flag == 1 && abs(temp) > 1
    out = 50e-6*cnt;  %0.0167 s : 360 deg => out ms : ? deg AND Ts_Control*cnt gives delta theta in time
    out = -2*pi*60*out;%(out*360*60)*(pi/180);
    if abs(out) > (180*pi/180)   % more than 180 deg is invalid! correct it with realistic logic later (with accurate capture of delay pulse)
        out = outOld;
    end
    flag = 0;
    cnt = 0;    
end

if flag == 0 && abs(temp) > 1
    flag = 1;
end

if flag == 1 && abs(temp) <= 1
    cnt = cnt +1;
end


outOld = out;
inOld = in;

== matlab function different_inverter_controls_BPS/GFM-VSG-100MW/FRT/In -RSY/grid health check logic V FRT/grid health ==
  settings: updateMethod=DISCRETE
  data: u input; y output; c input
function y = fcn(u,c)
persistent t1 cold1 cnt1 t2 cold2 cnt2 t3 cold3 cnt3 t4 cold4 cnt4 trip;
persistent t5 cold5 cnt5 t6 cold6 cnt6 t7 cold7 cnt7 t8 cold8 cnt8 t9 cold9 cnt9;

% % ITIC curve data
% lt = [0 0 0.02 0.02 0.5 0.5 10 10 100];20ms -> 0 V 500ms -> 70%; 
% lv = [0 0 0    70   70  80  80 90 90];  10s -> 80%; 100s -> 90%
% ut = [1e-3 3e-3 3e-3 0.5 0.5 100]; 1ms -> 200%; 3ms -> 140;
% uv = [200  140  120  120 110 110]; 500ms -> 120; 10s -> 110%

if isempty(t1)
    t1 = 0;
end
if isempty(cold1)
    cold1 = 0;
end
if isempty(cnt1)
    cnt1 = 0;
end
if isempty(t2)
    t2 = 0;
end
if isempty(cold2)
    cold2 = 0;
end
if isempty(cnt2)
    cnt2 = 0;
end
if isempty(t3)
    t3 = 0;
end
if isempty(cold3)
    cold3 = 0;
end
if isempty(cnt3)
    cnt3 = 0;
end
if isempty(t4)
    t4 = 0;
end
if isempty(cold4)
    cold4 = 0;
end
if isempty(cnt4)
    cnt4 = 0;
end
if isempty(t5)
    t5 = 0;
end
if isempty(cold5)
    cold5 = 0;
end
if isempty(cnt5)
    cnt5 = 0;
end
if isempty(t6)
    t6 = 0;
end
if isempty(cold6)
    cold6 = 0;
end
if isempty(cnt6)
    cnt6 = 0;
end
if isempty(t7)
    t7 = 0;
end
if isempty(cold7)
    cold7 = 0;
end
if isempty(cnt7)
    cnt7 = 0;
end
if isempty(t8)
    t8 = 0;
end
if isempty(cold8)
    cold8 = 0;
end
if isempty(cnt8)
    cnt8 = 0;
end
if isempty(t9)
    t9 = 0;
end
if isempty(cold9)
    cold9 = 0;
end
if isempty(cnt9)
    cnt9 = 0;
end
if isempty(trip)
    trip = 0;
end

%start health check after grid is stable after the simulation start
if (c > 1)
if(u(1)==0) %%if(u(1)==0 || u(2)==0 || u(3)==0 )
    if(cnt1==0)
    cnt1 = cnt1 +1;
    cold1 = c;     %start the new timer
    end
    t1 = c-cold1;  %lock the new timer
    if(t1>=0.16)
    trip = 1;      %timer exceeds ITIC limit
    end
else               %reset all variables
    cnt1 = 0;
    cold1 = 0;
    t1 = 0;
end


if(u(1)<=25) %%if(u(1)<=30 || u(2)<=30 || u(3)<=30)
    if(cnt2==0)
    cnt2 = cnt2 +1;
    cold2 = c;     %start the new timer
    end
    t2 = c-cold2;  %lock the new timer
    if(t2>=1.2)
    trip = 1;      %timer exceeds ITIC limit
    end
else               %reset all variables
    cnt2 = 0;
    cold2 = 0;
    t2 = 0;
end

if(u(1)<=50) %%if(u(1)<=50 || u(2)<=50 || u(3)<=50)
    if(cnt3==0)
    cnt3 = cnt3 +1;
    cold3 = c;     %start the new timer
    end
    t3 = c-cold3;  %lock the new timer
    if(t3>=2.5)      %%10s
    trip = 1;      %timer exceeds ITIC limit
    end
else               %reset all variables
    cnt3 = 0;
    cold3 = 0;
    t3 = 0;
end

if(u(1)<=70) %% if(u(1)<=80 || u(2)<=80 || u(3)<=80)
    if(cnt4==0)
    cnt4 = cnt4 +1;
    cold4 = c;     %start the new timer
    end
    t4 = c-cold4;  %lock the new timer
    if(t4>=3) %% 100s
    trip = 1;      %timer exceeds ITIC limit
    end
else               %reset all variables
    cnt4 = 0;
    cold4 = 0;
    t4 = 0;
end
% 
if(u(1)>=110) %%% if(u(1)<=85 || u(2)<=85 || u(3)<=85)
    if(cnt5==0)
    cnt5 = cnt5 +1;
    cold5 = c;     %start the new timer
    end
    t5 = c-cold5;  %lock the new timer
    if(t5>=1.2)
    trip = 1;      %timer exceeds ITIC limit
    end
else               %reset all variables
    cnt5 = 0;
    cold5 = 0;
    t5 = 0;
end
if(u(1)>=120) %%% if(u(1)>=200 || u(2)>=200 || u(3)>=200)
    if(cnt6==0)
    cnt6 = cnt6 +1;
    cold6 = c;     %start the new timer
    end
    t6 = c-cold6;  %lock the new timer
    if(t6>=0.16)
    trip = 1;      %timer exceeds ITIC limit
    end
else               %reset all variables
    cnt6 = 0;
    cold6 = 0;
    t6 = 0;
end

% 
% if(u>=140)
%     if(cnt6==0)
%     cnt6 = cnt6 +1;
%     cold6 = c;     %start the new timer
%     end
%     t6 = c-cold6;  %lock the new timer
%     if(t6>=0.003)
%     trip = 1;      %timer exceeds ITIC limit
%     end
% else               %reset all variables
%     cnt6 = 0;
%     cold6 = 0;
%     t6 = 0;
% end
% 
% if(u>=120)
%     if(cnt7==0)
%     cnt7 = cnt7 +1;
%     cold7 = c;     %start the new timer
%     end
%     t7 = c-cold7;  %lock the new timer
%     if(t7>=0.5)
%     trip = 1;      %timer exceeds ITIC limit
%     end
% else               %reset all variables
%     cnt7 = 0;
%     cold7 = 0;
%     t7 = 0;
% end
% % 
% if(u>=110)
%     if(cnt8==0)
%     cnt8 = cnt8 +1;
%     cold8 = c;     %start the new timer
%     end
%     t8 = c-cold8;  %lock the new timer
%     if(t8>=10)
%     trip = 1;      %timer exceeds ITIC limit
%     end
% else               %reset all variables
%     cnt8 = 0;
%     cold8 = 0;
%     t8 = 0;
% end

%clear trip if voltage is healthy for 100 ms
% if(trip == 1 && (u(1)>90&&u(2)>90&&u(3)>90) && (u(1)<110&&u(2)<110&&u(3)<110))
%     if(cnt9==0)
%     cnt9 = cnt9 +1;
%     cold9 = c;     %start the new timer
%     end
%     t9 = c-cold9;  %lock the new timer
%     if(t9>=0.1)
%     trip = 0;      %timer exceeds 100 ms reset trip
%     end
% else               %reset all variables
%     cnt9 = 0;
%     cold9 = 0;
%     t9 = 0;
% end
end

y = trip;

== matlab function different_inverter_controls_BPS/GFM-VSG-100MW/FRT/In -RSY/grid health check logic f FRT/grid health ==
  settings: updateMethod=DISCRETE
  data: u input; y output; c input
function y = fcn(u,c)
persistent t1 cold1 cnt1 t2 cold2 cnt2 t3 cold3 cnt3 t4 cold4 cnt4 trip;
persistent t5 cold5 cnt5 t6 cold6 cnt6 t7 cold7 cnt7 t8 cold8 cnt8 t9 cold9 cnt9;

% % ITIC curve data
% lt = [0 0 0.02 0.02 0.5 0.5 10 10 100];20ms -> 0 V 500ms -> 70%; 
% lv = [0 0 0    70   70  80  80 90 90];  10s -> 80%; 100s -> 90%
% ut = [1e-3 3e-3 3e-3 0.5 0.5 100]; 1ms -> 200%; 3ms -> 140;
% uv = [200  140  120  120 110 110]; 500ms -> 120; 10s -> 110%

if isempty(t1)
    t1 = 0;
end
if isempty(cold1)
    cold1 = 0;
end
if isempty(cnt1)
    cnt1 = 0;
end
if isempty(t2)
    t2 = 0;
end
if isempty(cold2)
    cold2 = 0;
end
if isempty(cnt2)
    cnt2 = 0;
end
if isempty(t3)
    t3 = 0;
end
if isempty(cold3)
    cold3 = 0;
end
if isempty(cnt3)
    cnt3 = 0;
end
if isempty(t4)
    t4 = 0;
end
if isempty(cold4)
    cold4 = 0;
end
if isempty(cnt4)
    cnt4 = 0;
end
if isempty(t5)
    t5 = 0;
end
if isempty(cold5)
    cold5 = 0;
end
if isempty(cnt5)
    cnt5 = 0;
end
if isempty(t6)
    t6 = 0;
end
if isempty(cold6)
    cold6 = 0;
end
if isempty(cnt6)
    cnt6 = 0;
end
if isempty(t7)
    t7 = 0;
end
if isempty(cold7)
    cold7 = 0;
end
if isempty(cnt7)
    cnt7 = 0;
end
if isempty(t8)
    t8 = 0;
end
if isempty(cold8)
    cold8 = 0;
end
if isempty(cnt8)
    cnt8 = 0;
end
if isempty(t9)
    t9 = 0;
end
if isempty(cold9)
    cold9 = 0;
end
if isempty(cnt9)
    cnt9 = 0;
end
if isempty(trip)
    trip = 0;
end

%start health check after grid is stable after the simulation start
if (c > 1)
    
if(u<=58.2 )
    if(cnt1==0)
    cnt1 = cnt1 +1;
    cold1 = c;     %start the new timer
    end
    t1 = c-cold1;  %lock the new timer
    if(t1>=299)
    trip = 1;      %timer exceeds ITIC limit
    end
else               %reset all variables
    cnt1 = 0;
    cold1 = 0;
    t1 = 0;
end


if(u>=63)
    if(cnt2==0)
    cnt2 = cnt2 +1;
    cold2 = c;     %start the new timer
    end
    t2 = c-cold2;  %lock the new timer
    if(t2>=299)
    trip = 1;      %timer exceeds ITIC limit
    end
else               %reset all variables
    cnt2 = 0;
    cold2 = 0;
    t2 = 0;
end
% 
% if(u<=58.2)
%     if(cnt3==0)
%     cnt3 = cnt3 +1;
%     cold3 = c;     %start the new timer
%     end
%     t3 = c-cold3;  %lock the new timer
%     if(t3>=299)
%     trip = 1;      %timer exceeds ITIC limit
%     end
% else               %reset all variables
%     cnt3 = 0;
%     cold3 = 0;
%     t3 = 0;
% end

% 
% if(u>=120)
%     if(cnt7==0)
%     cnt7 = cnt7 +1;
%     cold7 = c;     %start the new timer
%     end
%     t7 = c-cold7;  %lock the new timer
%     if(t7>=0.5)
%     trip = 1;      %timer exceeds ITIC limit
%     end
% else               %reset all variables
%     cnt7 = 0;
%     cold7 = 0;
%     t7 = 0;
% end
% 
% if(u>=110)
%     if(cnt8==0)
%     cnt8 = cnt8 +1;
%     cold8 = c;     %start the new timer
%     end
%     t8 = c-cold8;  %lock the new timer
%     if(t8>=10)
%     trip = 1;      %timer exceeds ITIC limit
%     end
% else               %reset all variables
%     cnt8 = 0;
%     cold8 = 0;
%     t8 = 0;
% end

%clear trip if voltage is healthy for 100 ms
% if(trip == 1 && (u(1)>90&&u(2)>90&&u(3)>90) && (u(1)<110&&u(2)<110&&u(3)<110))
%     if(cnt9==0)
%     cnt9 = cnt9 +1;
%     cold9 = c;     %start the new timer
%     end
%     t9 = c-cold9;  %lock the new timer
%     if(t9>=0.1)
%     trip = 0;      %timer exceeds 100 ms reset trip
%     end
% else               %reset all variables
%     cnt9 = 0;
%     cold9 = 0;
%     t9 = 0;
% end
end
y = trip;

== matlab function different_inverter_controls_BPS/GT-swing/Gen-a/Synchronous Machine G2 50 MVA 16.5 kV/ST6C EXCITER-1/MATLAB Function ==
  data: VTF input; u output; Vbias input
function u = fcn(VTF,Vbias)
%#codegen
if VTF > 1
    u=VTF;
    
else if VTF > Vbias
        u=1;
    else
        u=VTF/Vbias
    end
end
u;

== matlab function different_inverter_controls_BPS/GT-swing/Gen-a/Synchronous Machine G2 50 MVA 16.5 kV/ST6C EXCITER-1/MATLAB Function1 ==
  data: VT input; u output; QT input; PT input
function u = fcn(VT,QT,PT)
Xq=0.474;
Kadj= (((VT*VT)/Xq)+QT)/(sqrt(((((VT*VT)/Xq)+QT)*(((VT*VT)/Xq)+QT))+(PT*PT)))
u= Kadj;

== matlab function different_inverter_controls_BPS/GT-swing/Gen-a/Synchronous Machine G2 50 MVA 16.5 kV/ST6C EXCITER-1/MATLAB Function2 ==
  data: ISCLERR input; IOEX2 output; ISCLINV input; IUEX2 output
function [IOEX2,IUEX2] = fcn(ISCLERR,ISCLINV)
%#codegen

IOEX2= 0;
IUEX2= 0;

== matlab function different_inverter_controls_BPS/GFM-VSG-100MW/FRT/In -RSY/rising edge latch ==
  data: in input; out output
function out  = fcn(in)
    persistent n cnt
    if isempty(n)
        n = 0;
    end
    if isempty(cnt)
        cnt = 0;
    end
%start health check after grid is stable after the simulation start (1 s)
if (cnt > 20000)    
if n>0
    n = 1;
    out = 1;
else
    n = in;
    out = in;
end
else
    cnt = cnt +1;
    out = 0;
end

== matlab function different_inverter_controls_BPS/GFM-VSG-100MW/FRT/In -RSY/sync check logic/sync check ==
  settings: updateMethod=DISCRETE
  data: du input; df input; dth input; y output; tim input
function y = fcn(du,df,dth, tim)
persistent t1 con;

if isempty(con)
    con = 0;
end

if isempty(t1)
    t1 = 0;
end

if (tim > 11.9)
    if((abs(du(1)) < 0.05 && abs(du(2)) < 0.05 && abs(du(3)) < 0.05) && abs(df) < 0.04 && abs(dth) < 0.035)
        con = 1;
    end
end
y = con;

== matlab function different_inverter_controls_BPS/GFM-VSG-100MW/FRT/In -RSY/Latch ==
  data: u input; y output; c input
function y = fcn(u,c)
%#codegen
persistent tick started
if isempty(tick)
    tick = 0;
    started = 0;
end
y=0;
if u == 1 && c>1
    started = 1;
end
if started
    if tick<20000*6
        tick=tick+1;
        y = 1;
    else
        tick = 0;
        started = 0;
    end 
end
